simulink model "OAC_LA_Ass1_Task1_simu"  (R2018a)
settings: Solver=VariableStepAuto  StartTime=0.0  StopTime=10.0  RelTol=1e-3
values from neighbouring files (symbols this model uses):
  g = 9.81    [OAC_LA_Ass1.m]    (also in OAC_LA_Ass1_Task1.m; OAC_LA_Ass1_Task2.m)
  l = l_L1    [OAC_LA_Ass1.m]    (also in OAC_LA_Ass1_Task1.m = g/phat; OAC_LA_Ass1_Task2.m = 0.3; Task1_Funcs.m = g/phat)
  omega_0 = omega(1)    [OAC_LA_Ass1.m]    (also in OAC_LA_Ass1_Task1.m)
  phi_0 = phi(1)    [OAC_LA_Ass1.m]    (also in OAC_LA_Ass1_Task1.m)
settings Model: Creator=miko2  LastModifiedBy=miko2

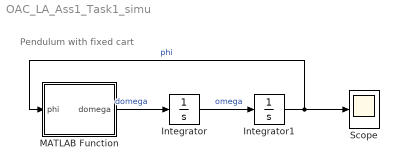
== system OAC_LA_Ass1_Task1_simu ==
  note: Pendulum with fixed cart
  Integrator : Integrator  InitialCondition=omega_0
  Integrator1 : Integrator  InitialCondition=phi_0
  MATLAB Function : MATLAB Function  TreatAsAtomicUnit=on
  Scope : Scope
  wires:
  MATLAB Function/1(domega) -> Integrator/1  "domega"
  Integrator/1 -> Integrator1/1  "omega"
  Integrator1/1 -> Scope/1, MATLAB Function/1(phi)  "phi"

== matlab function OAC_LA_Ass1_Task1_simu/MATLAB Function ==
  data: phi input size=3; domega output; g parameter; l parameter
function domega = fcn(phi,g, l)
    
    domega = g./ l .* sin(phi);
    
end
